simulink model "OneOneThrid"  (R2022b)
settings: Solver=VariableStepAuto  StartTime=0.0  StopTime=10.0  RelTol=1e-3
settings Model: Creator=yeyi5  LastModifiedBy=yeyi5
settings DataIOCC: ReturnWorkspaceOutputs=off

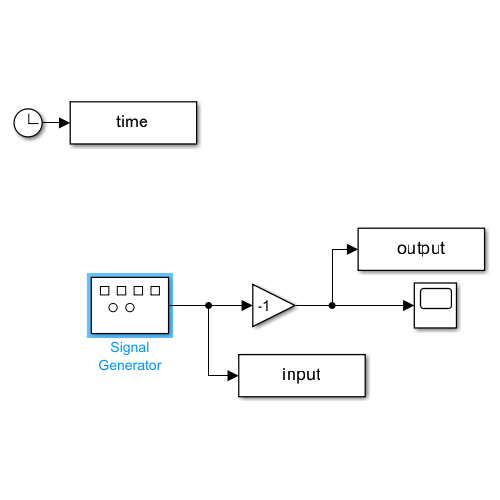
[thumbnail: Simulink's stored preview of the top-level diagram]
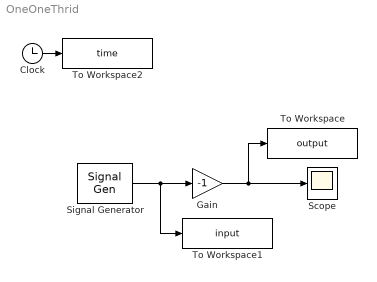
== system OneOneThrid ==
  Clock : Clock
  Gain : Gain  Gain=-1
  Scope : Scope
  Signal Generator : SignalGenerator  WaveForm=square  Amplitude=5  Frequency=5
  To Workspace : ToWorkspace  VariableName=output  SampleTime=-1
  To Workspace1 : ToWorkspace  VariableName=input  SampleTime=-1
  To Workspace2 : ToWorkspace  VariableName=time  SampleTime=-1
  wires:
  Clock/1 -> To Workspace2/1
  Gain/1 -> To Workspace/1, Scope/1
  Signal Generator/1 -> To Workspace1/1, Gain/1
